simulink model "lab_2_task"  (R2020a)
settings: Solver=VariableStepAuto  StartTime=0.0  StopTime=10.0  MaxStep=.01  RelTol=1e-3
settings Model: Creator=Administrator  LastModifiedBy=Administrator

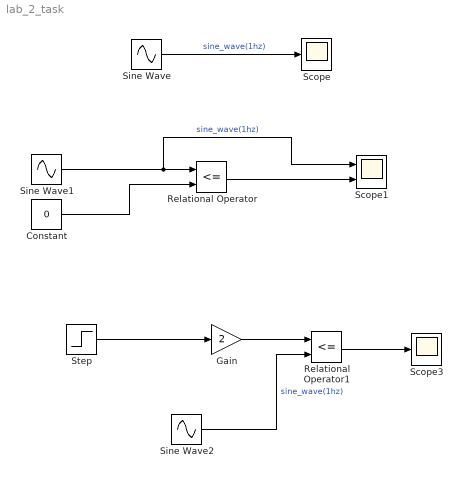
== system lab_2_task ==
  Constant : Constant  Value=0
  Gain : Gain  Gain=2
  Relational Operator : RelationalOperator  Operator=<=  OutDataTypeStr=boolean  RndMeth=Simplest
  Relational Operator1 : RelationalOperator  Operator=<=  OutDataTypeStr=boolean  RndMeth=Simplest
  Scope : Scope
  Scope1 : Scope  NumInputPorts=2
  Scope3 : Scope
  Sine Wave : Sin  Frequency=2*pi  SampleTime=0
  Sine Wave1 : Sin  Frequency=2*pi  SampleTime=0
  Sine Wave2 : Sin  Frequency=2*pi  SampleTime=0
  Step : Step  Time=2  SampleTime=0
  wires:
  Sine Wave/1 -> Scope/1  "sine_wave(1hz)"
  Sine Wave1/1 -> Scope1/1, Relational Operator/1  "sine_wave(1hz)"
  Constant/1 -> Relational Operator/2
  Relational Operator/1 -> Scope1/2
  Step/1 -> Gain/1
  Gain/1 -> Relational Operator1/1
  Sine Wave2/1 -> Relational Operator1/2  "sine_wave(1hz)"
  Relational Operator1/1 -> Scope3/1
